simulink library "FoldingMechanisms"  (R2017a)
settings: Solver=VariableStepAuto  StartTime=0.0  StopTime=10.0  RelTol=1e-3
undefined symbols (not defined in the file or in its folder): X, Y, Z
libraries: sm_lib x70, FoldingMechanisms x62, nesl_utility x7
(part 1 of 4)
settings Model: Creator=merz  LastModifiedBy=Paris

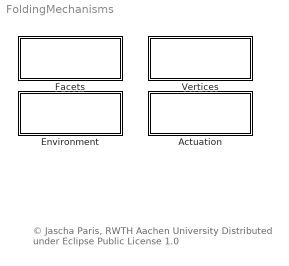
== system FoldingMechanisms ==
  note: © Jascha Paris, RWTH Aachen University
      |
      | Distributed under Eclipse Public License 1.0
  Actuation : Subsystem  Tag=FoldingMechanisms_sublibrary
      mask Display: disp(get_param(gcb,'Name'))
  Environment : Subsystem  Tag=FoldingMechanisms_sublibrary
      mask Display: disp(get_param(gcb,'Name'))
  Facets : Subsystem  Tag=FoldingMechanisms_sublibrary
      mask Display: disp(get_param(gcb,'Name'))
  Vertices : Subsystem  Tag=FoldingMechanisms_sublibrary
      mask Display: disp(get_param(gcb,'Name'))

== system FoldingMechanisms/Actuation ==
  Rotational Drive : Subsystem  mask{startang=1, endang=179, T_period=10, motion_select=sinus, forbac=on}
      mask prompts: startang "Start angle [°]"; endang "End angle [°]"; T_period "Periodic Time [s]"; motion_select "Motion Type"; forbac "Move forward and backward"
      mask init:
      | %Motion
      | startang_rad= startang*(pi/180);
      | endang_rad= endang*(pi/180);
      | steps=5000;
      | switch motion_select
      |     case 1
      |         t= [0,T_period/2]';
      |         y= [startang_rad,endang_rad]';
      |     case 2
      |         t= linspace(0,T_period/2,steps)';
      |         y= startang_rad+(endang_rad-startang_rad)*(1-(cos(linspace(0,pi,steps))'+1)/2);
      |     case 3
      |         t= linspace(0,T_period/2,steps)';
      |         z=t/(T_period/2);
      |         y=startang_rad+(endang_rad-startang_rad)*(6*z.^5-15*z.^4+10*z.^3);
      |     otherwise
      |         t= [0,T_period/2]';
      |         y= [startang_rad,endang_rad]';        
      | end
      | 
      | if (forbac==true)
      |     t= [t;t(2:end)+t(end)];
      |     y= [y;flipud(y(1:end-1))];    
      | end   
      |  
      | drivefunc = [t,y];
      mask TypeOptions motion_select: ramp | sinus | poly5
      mask DialogControl DescTextVar Prompt: This block provides, based on the parameters given below, a drive function for one foldangle of an actuated fold vertex
      mask Display:
      | plot([0.2 0.2], [0.2 0.8]);
      | plot([0.2 0.8], [0.2 0.2]);
      | 
      | scale_t=0.6/(max(t)-min(t));
      | scale_y=0.6/(max(y)-min(y));
      | 
      | plot(0.2+scale_t*(t-min(t)), 0.2+scale_y*(y-min(y)));

== system FoldingMechanisms/Environment ==
  Environment : Subsystem  Tag=simscape_sublibrary  mask{g_const=[0;0;-9.81]}
      mask prompts: g_const "Gravitational Constant"
      mask DialogControl DescTextVar Prompt: This Environment contains the local Simscape solver, gravity and the world coordinate system.
      mask Display: disp(get_param(gcb,'Name'))
  Options : Subsystem  Tag=simscape_sublibrary  mask{show3D=on}
      mask prompts: show3D "Show 3D Visualisation"
      mask Callback show3D:
      | show3D=get_param(gcb,'show3D');
      | mymodel=get_param(gcb,'parent');
      | if ~strcmp(mymodel,'FoldingMechanisms/Environment')
      |     if strcmp(show3D,'on');
      |         set_param(mymodel,'SimMechanicsOpenEditorOnUpdate','on');
      |     else
      |         set_param(mymodel,'SimMechanicsOpenEditorOnUpdate','off');
      |     end
      | end
      mask DialogControl DescTextVar Prompt: This block promotes options of the Simulation for convenience.
      mask Display: disp(get_param(gcb,'Name'))

== system FoldingMechanisms/Facets ==
  Piece of ellipsoid : Subsystem  Tag=simscape_sublibrary  mask{l1=0.4, l2=0.4, theta_x=35, tur1=off, tur2=off, t=0.01, clr=[200 200 200], tr=0.8, rjs1=on, rjs2=on, t_rj=0.01, cl_joint=[200 200 200]}
      mask prompts: l1 "Length S1 [m]"; l2 "Length S2 [m]"; theta_x "Angle alpha [°]"; tur1 "Turn COS at S1"; tur2 "Turn COS at S2"; t "Thickness [m]"; clr "Color RGB [3x1] with [0..255]"; tr "Transparency [0..1]"; rjs1 "at S1"; rjs2 "at S2"; t_rj "thickness"; cl_joint "Thickness [m]"
      mask init:
      | %Initialize Variables
      | a=0;
      | 
      | phi=linspace(0,theta_x,100);
      | r=linspace(l2,l1,100);
      | ellipsoid1=[r.*cosd(phi);r.*sind(phi)].';
      | 
      | %calculate geometry
      | cx=l1*cosd(theta_x);
      | cy=l1*sind(theta_x);
      | 
      | ellipsoid = [0 0; ellipsoid1];
      | 
      | bx=cx/2;
      | by=cy/2;
      | 
      | %Turn COS about 180° if enabled
      | turn1=0 + (tur1==true)*180;
      | turn2=0 + (tur2==true)*180;
      | 
      | %Convert color to vector with [0..1]
      | clr=clr/255;
      | cl_joint= cl_joint/255;
      | 
      | %Enable revolute joint visibility
      | %Convert logical to number
      | rj_true1=0 + (rjs1==true)*1;
      | rj_true2=0 + (rjs2==true)*1;
      mask DialogControl DescTextVar Prompt: Facet with two foldlines and an eliptic shape.
      mask DialogControl Container8 Prompt: Kinematic Dimensions
      mask DialogControl Container9 Prompt: Coordinate Systems
      mask DialogControl Control4 Prompt: Visualisation [on/off]
      mask Display:
      | %Geometry
      | X=[[0;0],ellipsoid1'];
      | 
      | %Normalized
      | dx=max(X(1,:))-min(X(1,:));
      | dy=max(X(2,:))-min(X(2,:));
      | dmax=max(dx,dy);
      | X=(X-[min(X(1,:));min(X(2,:))])/dmax*0.9+[0.05;0.05];
      | 
      | %Plot triangle
      | patch(X(1,:), X(2,:), clr);
      | plot([X(1,:),X(1,1)], [X(2,:),X(2,1)]);
      | 
      | 
      | %Labels in graphic
      | start_i=[1,1];
      | end_i=[size(X,2),2];
      | tur_f=[1,1];
      | 
      | color('blue');
      | for i=1:2
      |     if eval(['tur',num2str(i)])==tur_f(i)
      |         txt(i,1)='+';
      |         txt(i,2)='-';
      |     else
      |         txt(i,1)='-';
      |         txt(i,2)='+';
      |     end
      |     xs=X(1,start_i(i));
      |     vx=X(1,end_i(i))-X(1,start_i(i));
      |     ys=X(2,start_i(i));
      |     vy=X(2,end_i(i))-X(2,start_i(i));
      |     text(xs+vx*0.5,ys+vy*0.5,['S',num2str(i)]);
      |     text(xs+vx*0.3,ys+vy*0.3,txt(i,1));
      |     text(xs+vx*0.7,ys+vy*0.7,txt(i,2));
      | end
      | text((X(1,1)+X(1,end))/4,(X(2,1)+X(2,end))/7,'alpha');
  Quadrilateral : Subsystem  Tag=simscape_sublibrary  mask{l1=0.4, l2=0.4, l3=0.3, l4=0.5, alpha=80, tur1=off, tur2=off, tur3=off, tur4=off, t=0.01, clr=[200 200 200], tr=0.8, rjs1=on, rjs2=on, rjs3=on, rjs4=on, t_rj=0.01, cl_joint=[200 200 200]}
      mask prompts: l1 "Length S1 [m]"; l2 "Length S2 [m]"; l3 "Length S3 [m]"; l4 "Length S4 [m]"; alpha "Angle alpha [°]"; tur1 "Turn COS at S1"; tur2 "Turn COS at S2"; tur3 "Turn COS at S3"; tur4 "Turn COS at S4"; t "Thickness [m]"; clr "Color RGB [3x1] with [0..255]"; tr "Transparency [0..1]"; rjs1 "at S1"; rjs2 "at S2"; rjs3 "at S3"; rjs4 "at S4"; t_rj "Thickness [m]"; cl_joint "Color RGB [3x1] with [0..255]"
      mask init:
      | %Initialize Variables
      | a=0;
      | 
      | %calculate geometry
      | diagonal = sqrt(l1^2+l2^2-2*l1*l2*cosd(alpha));
      | 
      | a_x = 0;
      | a_y = 0;
      | b_x = l1*cosd(alpha);
      | b_y = l1*sind(alpha);
      | c_x = l2;
      | c_y = 0;
      | 
      | gamma1 = acosd((l2^2+diagonal^2-l1^2)/(2*l2*diagonal));
      | gamma2 = acosd((l3^2+diagonal^2-l4^2)/(2*l3*diagonal));
      | sigma = 180 - gamma1 - gamma2;
      | 
      | d_x = c_x + l3*cosd(sigma);
      | d_y = c_y + l3*sind(sigma);
      | 
      | ABmx = l1*cosd(alpha)/2;
      | ABmy = l1*sind(alpha)/2;
      | ACmx = l2/2;
      | ACmy = 0;
      | CDmx = c_x + l3*cosd(sigma)/2;
      | CDmy = c_y + l3*sind(sigma)/2;
      | 
      | beta1 = acosd((l1^2+diagonal^2-l2^2)/(2*l1*diagonal));
      | beta2 = acosd((l4^2+diagonal^2-l3^2)/(2*l4*diagonal));
      | epsilon = beta1 + beta2 + alpha - 180;
      | 
      | BDmx = b_x + l4*cosd(epsilon)/2;
      | BDmy = b_y + l4*sind(epsilon)/2;
      | 
      | quadrilateral=[b_x b_y; a_x a_y; c_x c_y; d_x d_y];
      | 
      | %Turn COS about 180° if enabled
      | turn1=0 + (tur1==true)*180;
      | turn2=0 + (tur2==true)*180;
      | turn3=0 + (tur3==true)*180;
      | turn4=0 + (tur4==true)*180;
      | 
      | %Convert color to vector with [0..1]
      | clr=clr/255;
      | cl_joint= cl_joint/255;
      | 
      | %Enable revolute joint visibility
      | %Convert logical to number
      | rj_true1=0 + (rjs1==true)*1;
      | rj_true2=0 + (rjs2==true)*1;
      | rj_true3=0 + (rjs3==true)*1;
      | rj_true4=0 + (rjs4==true)*1;
      mask DialogControl DescGroupVar Prompt: Quadrilateral Facet
      mask DialogControl DescTextVar Prompt: Facet with four foldlines.
      mask DialogControl Control3 Prompt: Visualisation [on/off]
      mask Display:
      | %Geometry
      | x_A=[a_x;a_y];
      | x_C=[c_x;c_y];
      | x_D=[d_x;d_y];
      | x_B=[b_x;b_y];
      | 
      | X=[x_A,x_C,x_D,x_B];
      | 
      | %Normalized
      | dx=max(X(1,:))-min(X(1,:));
      | dy=max(X(2,:))-min(X(2,:));
      | dmax=max(dx,dy);
      | X=(X-[min(X(1,:));min(X(2,:))])/dmax*0.9+[0.05;0.05];
      | 
      | %Plot Quadrilateral
      | patch(X(1,:), X(2,:), clr);
      | plot([X(1,:),X(1,1)], [X(2,:),X(2,1)]);
      | 
      | %Labels in graphic
      | color('blue');
      | 
      | start_i=[1,1,2,3];
      | end_i=[4,2,3,4];
      | tur_f=[1,1,1,0];
      | 
      | color('blue');
      | for i=1:4
      |     if eval(['tur',num2str(i)])==tur_f(i)
      |         txt(i,1)='+';
      |         txt(i,2)='-';
      |     else
      |         txt(i,1)='-';
      |         txt(i,2)='+';
      |     end
      |     xs=X(1,start_i(i));
      |     vx=X(1,end_i(i))-X(1,start_i(i));
      |     ys=X(2,start_i(i));
      |     vy=X(2,end_i(i))-X(2,start_i(i));
      |     text(xs+vx*0.5,ys+vy*0.5,['S',num2str(i)]);
      |     text(xs+vx*0.3,ys+vy*0.3,txt(i,1));
      |     text(xs+vx*0.7,ys+vy*0.7,txt(i,2));
      | end
      | text((X(1,1)+X(1,4))/4,(X(2,1)+X(2,4))/7,'alpha');
  Quintilateral : Subsystem  Tag=simscape_sublibrary  mask{l1=0.22, l2=0.13, l3=0.13, l4=0.27, l5=0.13, alpha=93, beta=120, tur1=off, tur2=off, tur3=off, tur4=off, tur5=off, thickness=0.01, clr=[200 200 200], tr=0.8, rjs1=on, rjs2=on, rjs3=on, rjs4=on, rjs5=on, t_rj=0.01, cl_joint=[200 200 200]}
      mask prompts: l1 "Length S1 [m]"; l2 "Length S2 [m]"; l3 "Length S3 [m]"; l4 "Length S4 [m]"; l5 "Length S5 [m]"; alpha "Angle alpha [°]"; beta "Angle beta [°]"; tur1 "Turn COS at S1"; tur2 "Turn COS at S2"; tur3 "Turn COS at S3"; tur4 "Turn COS at S4"; tur5 "Turn COS at S5"; thickness "Thickness [m]"; clr "Color RGB [3x1] with [0..255]"; tr "Transparency [0..1]"; rjs1 "at S1"; rjs2 "at S2"; rjs3 "at S3"; rjs4 "at S4"; rjs5 "at S5"; t_rj "Thickness [m]"; cl_joint "Color RGB [3x1] with [0..255]"
      mask init:
      | %Given Points
      | a_x = 0;
      | a_y = 0;
      | b_x = l2;
      | b_y = 0;
      | c_x = b_x+l3*cosd(180-beta);
      | c_y = b_y+l3*sind(180-beta);
      | e_x = l1*cosd(alpha);
      | e_y = l1*sind(alpha);
      | 
      | %calculate geometry
      | Dx=e_x-c_x;
      | Dy=e_y-c_y;
      | la=-l5;
      | lb=l4;
      | Calpha=(Dx^2+Dy^2+la^2-lb^2)/(2*la);
      | t=(Dy-sqrt(Dx^2+Dy^2-Calpha^2))/(Dx+Calpha);
      | talpha=2*atand(t);
      | Cbeta=(Dx^2+Dy^2+lb^2-la^2)/(2*lb);
      | tb=(Dy-sqrt(Dx^2+Dy^2-Cbeta^2))/(Dx+Cbeta);
      | tbeta=2*atand(tb);
      | d_x=e_x+(1-t^2)/(1+t^2)*l5;
      | d_y=e_y+(2*t)/(1+t^2)*l5;
      | 
      | quadrilateral=[a_x a_y; b_x b_y; c_x c_y; d_x d_y; e_x e_y];
      | 
      | %Turn COS about 180° if enabled
      | turn1=0 + (tur1==true)*180;
      | turn2=0 + (tur2==true)*180;
      | turn3=0 + (tur3==true)*180;
      | turn4=0 + (tur4==true)*180;
      | turn5=0 + (tur5==true)*180;
      | 
      | %Convert color to vector with [0..1]
      | clr=clr/255;
      | cl_joint= cl_joint/255;
      | 
      | %Enable revolute joint visibility
      | %Convert logical to number
      | rj_true1=0 + (rjs1==true)*1;
      | rj_true2=0 + (rjs2==true)*1;
      | rj_true3=0 + (rjs3==true)*1;
      | rj_true4=0 + (rjs4==true)*1;
      | rj_true5=0 + (rjs5==true)*1;
      mask DialogControl DescGroupVar Prompt: Quadrilateral Facet
      mask DialogControl DescTextVar Prompt: Facet with four foldlines.
      mask DialogControl Control3 Prompt: Visualisation [on/off]
      mask Display:
      | %Geometry
      | 
      | X=quadrilateral.';
      | 
      | %Normalized
      | dx=max(X(1,:))-min(X(1,:));
      | dy=max(X(2,:))-min(X(2,:));
      | dmax=max(dx,dy);
      | X=(X-[min(X(1,:));min(X(2,:))])/dmax*0.9+[0.05;0.05];
      | 
      | %Plot Quadrilateral
      | patch(X(1,:), X(2,:), clr);
      | plot([X(1,:),X(1,1)], [X(2,:),X(2,1)]);
      | 
      | 
      | %Labels in graphic
      | color('blue');
      | 
      | start_i=[1,1,2,3,4];
      | end_i=[5,2,3,4,5];
      | tur_f=[1,1,1,0,0];
      | 
      | color('blue');
      | for i=1:5
      |     if eval(['tur',num2str(i)])==tur_f(i)
      |         txt(i,1)='+';
      |         txt(i,2)='-';
      |     else
      |         txt(i,1)='-';
      |         txt(i,2)='+';
      |     end
      |     xs=X(1,start_i(i));
      |     vx=X(1,end_i(i))-X(1,start_i(i));
      |     ys=X(2,start_i(i));
      |     vy=X(2,end_i(i))-X(2,start_i(i));
      |     text(xs+vx*0.5,ys+vy*0.5,['S',num2str(i)]);
      |     text(xs+vx*0.3,ys+vy*0.3,txt(i,1));
      |     text(xs+vx*0.7,ys+vy*0.7,txt(i,2));
      | end
      | text((X(1,1)+X(1,2))/4,(X(2,1)+X(2,2))/2+0.06,'alpha');
      | text((X(1,1)+X(1,2))*3/4,(X(2,1)+X(2,2))/2+0.06,'beta');
  Triangle : Subsystem  Tag=simscape_sublibrary  mask{l1=0.4, l2=0.4, alpha=60, tur1=off, tur2=off, tur3=off, t=0.01, clr=[200 200 200], tr=0.8, rjs1=on, rjs2=on, rjs3=on, t_rj=0.01, cl_joint=[200 200 200]}
      mask prompts: l1 "Length S1 [m]"; l2 "Length S3 [m]"; alpha "Angle alpha [°]"; tur1 "Turn COS at S1"; tur2 "Turn COS at S2"; tur3 "Turn COS at S3"; t "Thickness [m]"; clr "Color RGB [3x1] with [0..255]"; tr "Transparency [0..1]"; rjs1 "at S1"; rjs2 "at S2"; rjs3 "at S3"; t_rj "Thickness [m]"; cl_joint "Color RGB [3x1] with [0..255]"
      mask init:
      | %Initialize Variables
      | a=0;
      | p=1;
      | 
      | %Calculate geometry
      | w1 = -l2/2 + l1*cosd(alpha);
      | h1 = p*(l1*sind(alpha));
      | l3 = sqrt(l1^2 + l2^2 - 2*l1*l2*cosd(alpha));
      | beta = acosd((l3^2+l2^2-l1^2)/(2*l3*l2));
      | w2 = -l2/2 + l1*cosd(alpha)/2;
      | w3 = l2/2 - l3*cosd(beta)/2;
      | h2 = (h1/2);
      | triangle= [w1 h1; p*(-l2/2) 0; p*(l2/2) 0];
      | 
      | %Turn COS about 180° if enabled
      | turn1=0 + (tur1==true)*180;
      | turn2=0 + (tur2==true)*180;
      | turn3=0 + (tur3==true)*180;
      | 
      | %Convert color to vector with [0..1]
      | clr=clr/255;
      | cl_joint= cl_joint/255;
      | 
      | %Enable revolute joint visibility
      | %Convert logical to number
      | rj_true1=0 + (rjs1==true)*1;
      | rj_true2=0 + (rjs2==true)*1;
      | rj_true3=0 + (rjs3==true)*1;
      mask DialogControl DescGroupVar Prompt: Triangular Facet
      mask DialogControl DescTextVar Prompt: Facet with three foldlines.
      mask DialogControl txt_rev Prompt: Visualisation [on/off]
      mask Display:
      | %Prepare visualisation of triangle
      | X=triangle';
      | 
      | %Normalize triangle
      | dx=max(X(1,:))-min(X(1,:));
      | dy=max(X(2,:))-min(X(2,:));
      | dmax=max(dx,dy);
      | X=(X-[min(X(1,:));min(X(2,:))])/dmax*0.9+[0.05;0.05];
      | 
      | %Plot triangle
      | patch(X(1,:), X(2,:), clr);
      | plot([X(1,:),X(1,1)], [X(2,:),X(2,1)]);
      | 
      | 
      | %Labels in graphic
      | 
      | start_i=[1,1,2];
      | end_i=[2,3,3];
      | tur_f=[0,0,1];
      | 
      | color('blue');
      | for i=1:3
      |     if eval(['tur',num2str(i)])==tur_f(i)
      |         txt(i,1)='+';
      |         txt(i,2)='-';
      |     else
      |         txt(i,1)='-';
      |         txt(i,2)='+';
      |     end
      |     xs=X(1,start_i(i));
      |     vx=X(1,end_i(i))-X(1,start_i(i));
      |     ys=X(2,start_i(i));
      |     vy=X(2,end_i(i))-X(2,start_i(i));
      |     text(xs+vx*0.5,ys+vy*0.5,['S',num2str(i)]);
      |     text(xs+vx*0.3,ys+vy*0.3,txt(i,1));
      |     text(xs+vx*0.7,ys+vy*0.7,txt(i,2));
      | end
      | text((X(1,1)+X(1,2))/4,(X(2,1)+X(2,2))/7,'alpha');

== system FoldingMechanisms/Vertices ==
  4-Foldlines Vertices : Subsystem  Tag=simscape_sublibrary
      mask Display: disp(get_param(gcb,'Name'))
  5-Foldlines Vertices : Subsystem  Tag=simscape_sublibrary
      mask Display: disp(get_param(gcb,'Name'))
  6-Foldlines Vertices : Subsystem  Tag=simscape_sublibrary
      mask Display: disp(get_param(gcb,'Name'))
  7-Foldlines Vertices : Subsystem  Tag=simscape_sublibrary
      mask Display: disp(get_param(gcb,'Name'))
  8-Foldlines Vertices : Subsystem  Tag=simscape_sublibrary
      mask Display: disp(get_param(gcb,'Name'))
  Subelements : Subsystem  Tag=simscape_sublibrary
      mask Display: disp(get_param(gcb,'Name'))

== system FoldingMechanisms/Actuation/Rotational Drive ==
  From Workspace : FromWorkspace  VariableName=drivefunc  SampleTime=0  OutputAfterFinalValue=Holding final value
  Drive Function : Outport
  wires:
  From Workspace/1 -> Drive Function/1

== system FoldingMechanisms/Environment/Environment ==
  Mechanism Configuration : sm_lib/Utilities/Mechanism Configuration  UniformGravity=Constant  GravityVector=g_const  GravityUnits=m/s^2  LinearizationDelta=0.001
  Solver Configuration : nesl_utility/Solver Configuration  PhysicalDomain=network_engine_domain  SubClassName=solver  LeftPortType=input  RightPortType=generic  Accelerate=off  Tones=[]  Harmonics=[]  SimulateNoise=off  Profile=off  UseLocalSampling=off  EnableSwitchedLinearOptims=on  FrequencyDomain=off  UseCCode=off  RelTol=0.001  AbsTol=1e-06  MinStep=1e-09  ToWorkspace=off  RevertToSquareIcSolve=off  NumHomotopyIterations=100  PhasorMode=off  PhasorModeNumHarmonics=1  OverrideAbsTol=off  DoDC=off  ResidualTolerance=1e-09  UseLocalSolver=off  LocalSolverChoice=NE_BACKWARD_EULER_ADVANCER  LocalSolverSampleTime=0.001  DoFixedCost=off  MaxNonlinIter=3  MaxModeIter=2  LinearAlgebra=Sparse  DelaysMemoryBudget=1024  AutomaticFiltering=on  FilteringTimeConstant=0.001
  World Frame : sm_lib/Frames and Transforms/World Frame
  Environment Port : PMIOPort  Port=1  Side=Right
  connections:
  Mechanism Configuration/RConn1 -- Environment Port/RConn1 -- World Frame/RConn1 -- Solver Configuration/RConn1

== system FoldingMechanisms/Environment/Options ==

== system FoldingMechanisms/Facets/Piece of ellipsoid ==
  Rigid Transform 1.1 : sm_lib/Frames and Transforms/Rigid Transform  TranslationMethod=Cartesian  TranslationStandardOffset=0  TranslationLengthUnit=m  TranslationStandardAxis=+Z  TranslationCartesianOffset=[bx by 0]  TranslationROffset=0  TranslationROffsetUnits=m  TranslationZOffset=0  TranslationZOffsetUnits=m  TranslationThetaOffset=0  TranslationThetaOffsetUnits=deg  RotationMethod=None  RotationAngleUnits=deg  RotationStandardAxis=+Z  RotationAngle=0.0  RotationArbitraryAxis=[0 0 1]  FollAlignAxisA=+X  BaseAlignAxisA=+Y  FollAlignAxisB=+Y  BaseAlignAxisB=+Z  RotationSequenceAxes=FollowerAxes  RotationSequence=XYX  RotationSequenceAngles=[0 0 0]  RotationSequenceAnglesUnits=deg  RotationMatrix=[1 0 0; 0 1 0; 0 0 1]
  Rigid Transform 1.2 : sm_lib/Frames and Transforms/Rigid Transform  TranslationMethod=None  TranslationStandardOffset=0  TranslationLengthUnit=m  TranslationStandardAxis=+Z  TranslationCartesianOffset=[0 0 0]  TranslationROffset=0  TranslationROffsetUnits=m  TranslationZOffset=0  TranslationZOffsetUnits=m  TranslationThetaOffset=0  TranslationThetaOffsetUnits=deg  RotationMethod=StandardAxis  RotationAngleUnits=deg  RotationStandardAxis=+Z  RotationAngle=theta_x  RotationArbitraryAxis=[0 0 1]  FollAlignAxisA=+X  BaseAlignAxisA=+Y  FollAlignAxisB=+Y  BaseAlignAxisB=+Z  RotationSequenceAxes=FollowerAxes  RotationSequence=XYX  RotationSequenceAngles=[0 0 0]  RotationSequenceAnglesUnits=deg  RotationMatrix=[1 0 0; 0 1 0; 0 0 1]
  Rigid Transform 1.3 : sm_lib/Frames and Transforms/Rigid Transform  TranslationMethod=None  TranslationStandardOffset=0  TranslationLengthUnit=m  TranslationStandardAxis=+Z  TranslationCartesianOffset=[0 0 0]  TranslationROffset=0  TranslationROffsetUnits=m  TranslationZOffset=0  TranslationZOffsetUnits=m  TranslationThetaOffset=0  TranslationThetaOffsetUnits=deg  RotationMethod=StandardAxis  RotationAngleUnits=deg  RotationStandardAxis=+Y  RotationAngle=90  RotationArbitraryAxis=[0 0 1]  FollAlignAxisA=+X  BaseAlignAxisA=+Y  FollAlignAxisB=+Y  BaseAlignAxisB=+Z  RotationSequenceAxes=FollowerAxes  RotationSequence=XYX  RotationSequenceAngles=[0 0 0]  RotationSequenceAnglesUnits=deg  RotationMatrix=[1 0 0; 0 1 0; 0 0 1]
  Rigid Transform 1.4 : sm_lib/Frames and Transforms/Rigid Transform  TranslationMethod=None  TranslationStandardOffset=0  TranslationLengthUnit=m  TranslationStandardAxis=+Z  TranslationCartesianOffset=[0 0 0]  TranslationROffset=0  TranslationROffsetUnits=m  TranslationZOffset=0  TranslationZOffsetUnits=m  TranslationThetaOffset=0  TranslationThetaOffsetUnits=deg  RotationMethod=StandardAxis  RotationAngleUnits=deg  RotationStandardAxis=+X  RotationAngle=turn1  RotationArbitraryAxis=[0 0 1]  FollAlignAxisA=+X  BaseAlignAxisA=+Y  FollAlignAxisB=+Y  BaseAlignAxisB=+Z  RotationSequenceAxes=FollowerAxes  RotationSequence=XYX  RotationSequenceAngles=[0 0 0]  RotationSequenceAnglesUnits=deg  RotationMatrix=[1 0 0; 0 1 0; 0 0 1]
  Rigid Transform 2.1 : sm_lib/Frames and Transforms/Rigid Transform  TranslationMethod=Cartesian  TranslationStandardOffset=0  TranslationLengthUnit=m  TranslationStandardAxis=+Z  TranslationCartesianOffset=[l2/2 0 0]  TranslationROffset=0  TranslationROffsetUnits=m  TranslationZOffset=0  TranslationZOffsetUnits=m  TranslationThetaOffset=0  TranslationThetaOffsetUnits=deg  RotationMethod=StandardAxis  RotationAngleUnits=deg  RotationStandardAxis=+Y  RotationAngle=90  RotationArbitraryAxis=[0 0 1]  FollAlignAxisA=+X  BaseAlignAxisA=+Y  FollAlignAxisB=+Y  BaseAlignAxisB=+Z  RotationSequenceAxes=FollowerAxes  RotationSequence=XYX  RotationSequenceAngles=[0 0 0]  RotationSequenceAnglesUnits=deg  RotationMatrix=[1 0 0; 0 1 0; 0 0 1]
  Rigid Transform 2.2 : sm_lib/Frames and Transforms/Rigid Transform  TranslationMethod=None  TranslationStandardOffset=0  TranslationLengthUnit=m  TranslationStandardAxis=+Z  TranslationCartesianOffset=[0 0 0]  TranslationROffset=0  TranslationROffsetUnits=m  TranslationZOffset=0  TranslationZOffsetUnits=m  TranslationThetaOffset=0  TranslationThetaOffsetUnits=deg  RotationMethod=StandardAxis  RotationAngleUnits=deg  RotationStandardAxis=+X  RotationAngle=turn2  RotationArbitraryAxis=[0 0 1]  FollAlignAxisA=+X  BaseAlignAxisA=+Y  FollAlignAxisB=+Y  BaseAlignAxisB=+Z  RotationSequenceAxes=FollowerAxes  RotationSequence=XYX  RotationSequenceAngles=[0 0 0]  RotationSequenceAnglesUnits=deg  RotationMatrix=[1 0 0; 0 1 0; 0 0 1]
  Solid_RJ1 : sm_lib/Body Elements/Solid  InertiaType=PointMass  Mass=0  MassUnits=kg  CenterOfMass=[0 0 0]  CenterOfMassUnits=m  MomentsOfInertia=[1 1 1]  MomentsOfInertiaUnits=kg*m^2  ProductsOfInertia=[1 1 1]  ProductsOfInertiaUnits=kg*m^2  DensityBased=on  Density=1000  DensityUnits=kg/m^3  DoExposeReferenceFrame=off  SerializedFrames=<Frames><Frame><Id>Frame1</Id><Value><Name>S1</Name><Origin><Source>ReferenceFrame</Source><FeatureName></FeatureName></Origin><PrimaryAxis><DefinedDirection>+Z</DefinedDirection><Source>ReferenceFrame</Source><SourceDirection>+Z</SourceDirection><FeatureName></FeatureName></PrimaryAxis><SecondaryAxis><DefinedDirection>+X</DefinedDirection><Source>ReferenceFrame</Source><SourceDirection>+X</SourceDirection><FeatureName></FeatureName></SecondaryAxis></Value></Frame></Frames>  GraphicType=FromGeometry  MarkerShape=Sphere  MarkerSize=10  GraphicVisPropType=SimpleVisualProperties  GraphicDiffuseColor=cl_joint  GraphicSpecularColor=[0.5 0.5 0.5 1.0]  GraphicAmbientColor=[0.15 0.15 0.15 1.0]  GraphicEmissiveColor=[0.0 0.0 0.0 1.0]  GraphicShininess=75  GraphicOpacity=rj_true1  GeometryShape=Cylinder  RectangleSize=[1 1]  RectangleSizeUnits=m  BrickDimensions=[1 1 1]  BrickDimensionUnits=m  CylinderRadius=t_rj  CylinderRadiusUnits=m  CylinderLength=l1  CylinderLengthUnits=m  SphereRadius=1  SphereRadiusUnits=m  EllipsoidRadii=[1 1 1]  EllipsoidRadiiUnits=m  ExtrusionCrossSection=[1 1; -1 1; -1 -1; 1 -1]  ExtrusionCrossSectionUnits=m  ExtrusionLength=1  ExtrusionLengthUnits=m  PolygonNumSides=3  PolygonOuterRadius=1  PolygonOuterRadiusUnits=m  ExtGeomFileType=STEP  ExtGeomFileUnits=m  RevolutionCrossSection=[1 1; 1 -1; 2 -1; 2 1]  RevolutionCrossSectionUnits=m  RevolutionExtent=Full  RevolutionAngle=180  RevolutionAngleUnits=deg
  Solid_RJ2 : sm_lib/Body Elements/Solid  InertiaType=PointMass  Mass=0  MassUnits=kg  CenterOfMass=[0 0 0]  CenterOfMassUnits=m  MomentsOfInertia=[1 1 1]  MomentsOfInertiaUnits=kg*m^2  ProductsOfInertia=[1 1 1]  ProductsOfInertiaUnits=kg*m^2  DensityBased=on  Density=1000  DensityUnits=kg/m^3  DoExposeReferenceFrame=off  SerializedFrames=<Frames><Frame><Id>Frame1</Id><Value><Name>S2</Name><Origin><Source>ReferenceFrame</Source><FeatureName></FeatureName></Origin><PrimaryAxis><DefinedDirection>+Z</DefinedDirection><Source>ReferenceFrame</Source><SourceDirection>+Z</SourceDirection><FeatureName></FeatureName></PrimaryAxis><SecondaryAxis><DefinedDirection>+X</DefinedDirection><Source>ReferenceFrame</Source><SourceDirection>+X</SourceDirection><FeatureName></FeatureName></SecondaryAxis></Value></Frame></Frames>  GraphicType=FromGeometry  MarkerShape=Sphere  MarkerSize=10  GraphicVisPropType=SimpleVisualProperties  GraphicDiffuseColor=cl_joint  GraphicSpecularColor=[0.5 0.5 0.5 1.0]  GraphicAmbientColor=[0.15 0.15 0.15 1.0]  GraphicEmissiveColor=[0.0 0.0 0.0 1.0]  GraphicShininess=75  GraphicOpacity=rj_true2  GeometryShape=Cylinder  RectangleSize=[1 1]  RectangleSizeUnits=m  BrickDimensions=[1 1 1]  BrickDimensionUnits=m  CylinderRadius=t_rj  CylinderRadiusUnits=m  CylinderLength=l2  CylinderLengthUnits=m  SphereRadius=1  SphereRadiusUnits=m  EllipsoidRadii=[1 1 1]  EllipsoidRadiiUnits=m  ExtrusionCrossSection=[1 1; -1 1; -1 -1; 1 -1]  ExtrusionCrossSectionUnits=m  ExtrusionLength=1  ExtrusionLengthUnits=m  PolygonNumSides=3  PolygonOuterRadius=1  PolygonOuterRadiusUnits=m  ExtGeomFileType=STEP  ExtGeomFileUnits=m  RevolutionCrossSection=[1 1; 1 -1; 2 -1; 2 1]  RevolutionCrossSectionUnits=m  RevolutionExtent=Full  RevolutionAngle=180  RevolutionAngleUnits=deg
  Solid_ellipsoid : sm_lib/Body Elements/Solid  InertiaType=CalculateFromGeometry  Mass=1  MassUnits=kg  CenterOfMass=[0 0 0]  CenterOfMassUnits=m  MomentsOfInertia=[1 1 1]  MomentsOfInertiaUnits=kg*m^2  ProductsOfInertia=[1 1 1]  ProductsOfInertiaUnits=kg*m^2  DensityBased=on  Density=1000  DensityUnits=kg/m^3  DoExposeReferenceFrame=on  SerializedFrames=<Frames/>  GraphicType=FromGeometry  MarkerShape=Sphere  MarkerSize=10  GraphicVisPropType=SimpleVisualProperties  GraphicDiffuseColor=clr  GraphicSpecularColor=[0.5 0.5 0.5 1.0]  GraphicAmbientColor=[0.15 0.15 0.15 1.0]  GraphicEmissiveColor=[0.0 0.0 0.0 1.0]  GraphicShininess=75  GraphicOpacity=tr  GeometryShape=GeneralExtrusion  RectangleSize=[1 1]  RectangleSizeUnits=m  BrickDimensions=[1 1 1]  BrickDimensionUnits=m  CylinderRadius=1  CylinderRadiusUnits=m  CylinderLength=1  CylinderLengthUnits=m  SphereRadius=1  SphereRadiusUnits=m  EllipsoidRadii=[1 1 1]  EllipsoidRadiiUnits=m  ExtrusionCrossSection=ellipsoid  ExtrusionCrossSectionUnits=m  ExtrusionLength=t  ExtrusionLengthUnits=m  PolygonNumSides=3  PolygonOuterRadius=1  PolygonOuterRadiusUnits=m  ExtGeomFileType=STEP  ExtGeomFileUnits=m  RevolutionCrossSection=[1 1; 1 -1; 2 -1; 2 1]  RevolutionCrossSectionUnits=m  RevolutionExtent=Full  RevolutionAngle=180  RevolutionAngleUnits=deg
  S1 : PMIOPort  Port=1  Side=Left
  S2 : PMIOPort  Port=2  Side=Right
  connections:
  Rigid Transform 2.2/LConn1 -- Rigid Transform 2.1/RConn1
  Rigid Transform 1.3/RConn1 -- Rigid Transform 1.4/LConn1
  Rigid Transform 1.3/LConn1 -- Rigid Transform 1.2/RConn1
  Rigid Transform 1.2/LConn1 -- Rigid Transform 1.1/RConn1
  Solid_ellipsoid/RConn1 -- Rigid Transform 2.1/LConn1 -- Rigid Transform 1.1/LConn1
  S2/RConn1 -- Solid_RJ2/LConn1 -- Rigid Transform 2.2/RConn1
  S1/RConn1 -- Solid_RJ1/LConn1 -- Rigid Transform 1.4/RConn1

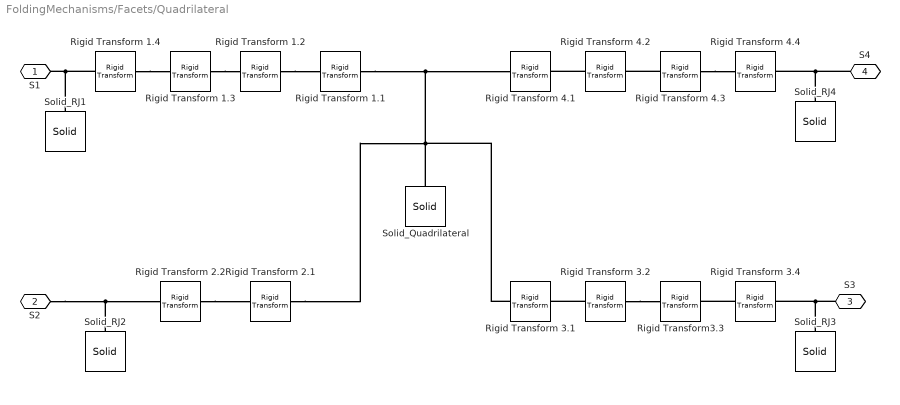
== system FoldingMechanisms/Facets/Quadrilateral ==
  Rigid Transform 1.1 : sm_lib/Frames and Transforms/Rigid Transform  TranslationMethod=Cartesian  TranslationStandardOffset=0  TranslationLengthUnit=m  TranslationStandardAxis=+Z  TranslationCartesianOffset=[ABmx ABmy 0]  TranslationROffset=0  TranslationROffsetUnits=m  TranslationZOffset=0  TranslationZOffsetUnits=m  TranslationThetaOffset=0  TranslationThetaOffsetUnits=deg  RotationMethod=None  RotationAngleUnits=deg  RotationStandardAxis=+Z  RotationAngle=0.0  RotationArbitraryAxis=[0 0 1]  FollAlignAxisA=+X  BaseAlignAxisA=+Y  FollAlignAxisB=+Y  BaseAlignAxisB=+Z  RotationSequenceAxes=FollowerAxes  RotationSequence=XYX  RotationSequenceAngles=[0 0 0]  RotationSequenceAnglesUnits=deg  RotationMatrix=[1 0 0; 0 1 0; 0 0 1]
  Rigid Transform 1.2 : sm_lib/Frames and Transforms/Rigid Transform  TranslationMethod=None  TranslationStandardOffset=0  TranslationLengthUnit=m  TranslationStandardAxis=+Z  TranslationCartesianOffset=[0 0 0]  TranslationROffset=0  TranslationROffsetUnits=m  TranslationZOffset=0  TranslationZOffsetUnits=m  TranslationThetaOffset=0  TranslationThetaOffsetUnits=deg  RotationMethod=StandardAxis  RotationAngleUnits=deg  RotationStandardAxis=+Z  RotationAngle=alpha  RotationArbitraryAxis=[0 0 1]  FollAlignAxisA=+X  BaseAlignAxisA=+Y  FollAlignAxisB=+Y  BaseAlignAxisB=+Z  RotationSequenceAxes=FollowerAxes  RotationSequence=XYX  RotationSequenceAngles=[0 0 0]  RotationSequenceAnglesUnits=deg  RotationMatrix=[1 0 0; 0 1 0; 0 0 1]
  Rigid Transform 1.3 : sm_lib/Frames and Transforms/Rigid Transform  TranslationMethod=Cartesian  TranslationStandardOffset=0  TranslationLengthUnit=m  TranslationStandardAxis=+Z  TranslationCartesianOffset=[0 a 0]  TranslationROffset=0  TranslationROffsetUnits=m  TranslationZOffset=0  TranslationZOffsetUnits=m  TranslationThetaOffset=0  TranslationThetaOffsetUnits=deg  RotationMethod=StandardAxis  RotationAngleUnits=deg  RotationStandardAxis=+Y  RotationAngle=90  RotationArbitraryAxis=[0 0 1]  FollAlignAxisA=+X  BaseAlignAxisA=+Y  FollAlignAxisB=+Y  BaseAlignAxisB=+Z  RotationSequenceAxes=FollowerAxes  RotationSequence=XYX  RotationSequenceAngles=[0 0 0]  RotationSequenceAnglesUnits=deg  RotationMatrix=[1 0 0; 0 1 0; 0 0 1]
  Rigid Transform 1.4 : sm_lib/Frames and Transforms/Rigid Transform  TranslationMethod=None  TranslationStandardOffset=0  TranslationLengthUnit=m  TranslationStandardAxis=+Z  TranslationCartesianOffset=[0 0 0]  TranslationROffset=0  TranslationROffsetUnits=m  TranslationZOffset=0  TranslationZOffsetUnits=m  TranslationThetaOffset=0  TranslationThetaOffsetUnits=deg  RotationMethod=StandardAxis  RotationAngleUnits=deg  RotationStandardAxis=+X  RotationAngle=turn1  RotationArbitraryAxis=[0 0 1]  FollAlignAxisA=+X  BaseAlignAxisA=+Y  FollAlignAxisB=+Y  BaseAlignAxisB=+Z  RotationSequenceAxes=FollowerAxes  RotationSequence=XYX  RotationSequenceAngles=[0 0 0]  RotationSequenceAnglesUnits=deg  RotationMatrix=[1 0 0; 0 1 0; 0 0 1]
  Rigid Transform 2.1 : sm_lib/Frames and Transforms/Rigid Transform  TranslationMethod=Cartesian  TranslationStandardOffset=0  TranslationLengthUnit=m  TranslationStandardAxis=+Z  TranslationCartesianOffset=[ACmx ACmy 0]  TranslationROffset=0  TranslationROffsetUnits=m  TranslationZOffset=0  TranslationZOffsetUnits=m  TranslationThetaOffset=0  TranslationThetaOffsetUnits=deg  RotationMethod=StandardAxis  RotationAngleUnits=deg  RotationStandardAxis=+Y  RotationAngle=90  RotationArbitraryAxis=[0 0 1]  FollAlignAxisA=+X  BaseAlignAxisA=+Y  FollAlignAxisB=+Y  BaseAlignAxisB=+Z  RotationSequenceAxes=FollowerAxes  RotationSequence=XYX  RotationSequenceAngles=[0 0 0]  RotationSequenceAnglesUnits=deg  RotationMatrix=[1 0 0; 0 1 0; 0 0 1]
  Rigid Transform 2.2 : sm_lib/Frames and Transforms/Rigid Transform  TranslationMethod=None  TranslationStandardOffset=0  TranslationLengthUnit=m  TranslationStandardAxis=+Z  TranslationCartesianOffset=[0 0 0]  TranslationROffset=0  TranslationROffsetUnits=m  TranslationZOffset=0  TranslationZOffsetUnits=m  TranslationThetaOffset=0  TranslationThetaOffsetUnits=deg  RotationMethod=StandardAxis  RotationAngleUnits=deg  RotationStandardAxis=+X  RotationAngle=turn2  RotationArbitraryAxis=[0 0 1]  FollAlignAxisA=+X  BaseAlignAxisA=+Y  FollAlignAxisB=+Y  BaseAlignAxisB=+Z  RotationSequenceAxes=FollowerAxes  RotationSequence=XYX  RotationSequenceAngles=[0 0 0]  RotationSequenceAnglesUnits=deg  RotationMatrix=[1 0 0; 0 1 0; 0 0 1]
  Rigid Transform 3.1 : sm_lib/Frames and Transforms/Rigid Transform  TranslationMethod=Cartesian  TranslationStandardOffset=0  TranslationLengthUnit=m  TranslationStandardAxis=+Z  TranslationCartesianOffset=[CDmx CDmy 0]  TranslationROffset=0  TranslationROffsetUnits=m  TranslationZOffset=0  TranslationZOffsetUnits=m  TranslationThetaOffset=0  TranslationThetaOffsetUnits=deg  RotationMethod=None  RotationAngleUnits=deg  RotationStandardAxis=+Z  RotationAngle=0.0  RotationArbitraryAxis=[0 0 1]  FollAlignAxisA=+X  BaseAlignAxisA=+Y  FollAlignAxisB=+Y  BaseAlignAxisB=+Z  RotationSequenceAxes=FollowerAxes  RotationSequence=XYX  RotationSequenceAngles=[0 0 0]  RotationSequenceAnglesUnits=deg  RotationMatrix=[1 0 0; 0 1 0; 0 0 1]
  Rigid Transform 3.2 : sm_lib/Frames and Transforms/Rigid Transform  TranslationMethod=None  TranslationStandardOffset=0  TranslationLengthUnit=m  TranslationStandardAxis=+Z  TranslationCartesianOffset=[0 0 0]  TranslationROffset=0  TranslationROffsetUnits=m  TranslationZOffset=0  TranslationZOffsetUnits=m  TranslationThetaOffset=0  TranslationThetaOffsetUnits=deg  RotationMethod=StandardAxis  RotationAngleUnits=deg  RotationStandardAxis=+Z  RotationAngle=sigma  RotationArbitraryAxis=[0 0 1]  FollAlignAxisA=+X  BaseAlignAxisA=+Y  FollAlignAxisB=+Y  BaseAlignAxisB=+Z  RotationSequenceAxes=FollowerAxes  RotationSequence=XYX  RotationSequenceAngles=[0 0 0]  RotationSequenceAnglesUnits=deg  RotationMatrix=[1 0 0; 0 1 0; 0 0 1]
  Rigid Transform 3.4 : sm_lib/Frames and Transforms/Rigid Transform  TranslationMethod=None  TranslationStandardOffset=0  TranslationLengthUnit=m  TranslationStandardAxis=+Z  TranslationCartesianOffset=[0 0 0]  TranslationROffset=0  TranslationROffsetUnits=m  TranslationZOffset=0  TranslationZOffsetUnits=m  TranslationThetaOffset=0  TranslationThetaOffsetUnits=deg  RotationMethod=StandardAxis  RotationAngleUnits=deg  RotationStandardAxis=+X  RotationAngle=turn3  RotationArbitraryAxis=[0 0 1]  FollAlignAxisA=+X  BaseAlignAxisA=+Y  FollAlignAxisB=+Y  BaseAlignAxisB=+Z  RotationSequenceAxes=FollowerAxes  RotationSequence=XYX  RotationSequenceAngles=[0 0 0]  RotationSequenceAnglesUnits=deg  RotationMatrix=[1 0 0; 0 1 0; 0 0 1]
  Rigid Transform 4.1 : sm_lib/Frames and Transforms/Rigid Transform  TranslationMethod=Cartesian  TranslationStandardOffset=0  TranslationLengthUnit=m  TranslationStandardAxis=+Z  TranslationCartesianOffset=[BDmx BDmy 0]  TranslationROffset=0  TranslationROffsetUnits=m  TranslationZOffset=0  TranslationZOffsetUnits=m  TranslationThetaOffset=0  TranslationThetaOffsetUnits=deg  RotationMethod=None  RotationAngleUnits=deg  RotationStandardAxis=+Z  RotationAngle=0.0  RotationArbitraryAxis=[0 0 1]  FollAlignAxisA=+X  BaseAlignAxisA=+Y  FollAlignAxisB=+Y  BaseAlignAxisB=+Z  RotationSequenceAxes=FollowerAxes  RotationSequence=XYX  RotationSequenceAngles=[0 0 0]  RotationSequenceAnglesUnits=deg  RotationMatrix=[1 0 0; 0 1 0; 0 0 1]
  Rigid Transform 4.2 : sm_lib/Frames and Transforms/Rigid Transform  TranslationMethod=None  TranslationStandardOffset=0  TranslationLengthUnit=m  TranslationStandardAxis=+Z  TranslationCartesianOffset=[0 0 0]  TranslationROffset=0  TranslationROffsetUnits=m  TranslationZOffset=0  TranslationZOffsetUnits=m  TranslationThetaOffset=0  TranslationThetaOffsetUnits=deg  RotationMethod=StandardAxis  RotationAngleUnits=deg  RotationStandardAxis=+Z  RotationAngle=epsilon  RotationArbitraryAxis=[0 0 1]  FollAlignAxisA=+X  BaseAlignAxisA=+Y  FollAlignAxisB=+Y  BaseAlignAxisB=+Z  RotationSequenceAxes=FollowerAxes  RotationSequence=XYX  RotationSequenceAngles=[0 0 0]  RotationSequenceAnglesUnits=deg  RotationMatrix=[1 0 0; 0 1 0; 0 0 1]
  Rigid Transform 4.3 : sm_lib/Frames and Transforms/Rigid Transform  TranslationMethod=Cartesian  TranslationStandardOffset=0  TranslationLengthUnit=m  TranslationStandardAxis=+Z  TranslationCartesianOffset=[0 -a 0]  TranslationROffset=0  TranslationROffsetUnits=m  TranslationZOffset=0  TranslationZOffsetUnits=m  TranslationThetaOffset=0  TranslationThetaOffsetUnits=deg  RotationMethod=StandardAxis  RotationAngleUnits=deg  RotationStandardAxis=+Y  RotationAngle=90  RotationArbitraryAxis=[0 0 1]  FollAlignAxisA=+X  BaseAlignAxisA=+Y  FollAlignAxisB=+Y  BaseAlignAxisB=+Z  RotationSequenceAxes=FollowerAxes  RotationSequence=XYX  RotationSequenceAngles=[0 0 0]  RotationSequenceAnglesUnits=deg  RotationMatrix=[1 0 0; 0 1 0; 0 0 1]
  Rigid Transform 4.4 : sm_lib/Frames and Transforms/Rigid Transform  TranslationMethod=None  TranslationStandardOffset=0  TranslationLengthUnit=m  TranslationStandardAxis=+Z  TranslationCartesianOffset=[0 0 0]  TranslationROffset=0  TranslationROffsetUnits=m  TranslationZOffset=0  TranslationZOffsetUnits=m  TranslationThetaOffset=0  TranslationThetaOffsetUnits=deg  RotationMethod=StandardAxis  RotationAngleUnits=deg  RotationStandardAxis=+X  RotationAngle=turn4  RotationArbitraryAxis=[0 0 1]  FollAlignAxisA=+X  BaseAlignAxisA=+Y  FollAlignAxisB=+Y  BaseAlignAxisB=+Z  RotationSequenceAxes=FollowerAxes  RotationSequence=XYX  RotationSequenceAngles=[0 0 0]  RotationSequenceAnglesUnits=deg  RotationMatrix=[1 0 0; 0 1 0; 0 0 1]
  Rigid Transform3.3 : sm_lib/Frames and Transforms/Rigid Transform  TranslationMethod=Cartesian  TranslationStandardOffset=0  TranslationLengthUnit=m  TranslationStandardAxis=+Z  TranslationCartesianOffset=[0 a 0]  TranslationROffset=0  TranslationROffsetUnits=m  TranslationZOffset=0  TranslationZOffsetUnits=m  TranslationThetaOffset=0  TranslationThetaOffsetUnits=deg  RotationMethod=StandardAxis  RotationAngleUnits=deg  RotationStandardAxis=+Y  RotationAngle=90  RotationArbitraryAxis=[0 0 1]  FollAlignAxisA=+X  BaseAlignAxisA=+Y  FollAlignAxisB=+Y  BaseAlignAxisB=+Z  RotationSequenceAxes=FollowerAxes  RotationSequence=XYX  RotationSequenceAngles=[0 0 0]  RotationSequenceAnglesUnits=deg  RotationMatrix=[1 0 0; 0 1 0; 0 0 1]
  Solid_Quadrilateral : sm_lib/Body Elements/Solid  InertiaType=CalculateFromGeometry  Mass=1  MassUnits=kg  CenterOfMass=[0 0 0]  CenterOfMassUnits=m  MomentsOfInertia=[1 1 1]  MomentsOfInertiaUnits=kg*m^2  ProductsOfInertia=[1 1 1]  ProductsOfInertiaUnits=kg*m^2  DensityBased=on  Density=1000  DensityUnits=kg/m^3  DoExposeReferenceFrame=on  SerializedFrames=<Frames/>  GraphicType=FromGeometry  MarkerShape=Sphere  MarkerSize=10  GraphicVisPropType=SimpleVisualProperties  GraphicDiffuseColor=clr  GraphicSpecularColor=[0.5 0.5 0.5 1.0]  GraphicAmbientColor=[0.15 0.15 0.15 1.0]  GraphicEmissiveColor=[0.0 0.0 0.0 1.0]  GraphicShininess=75  GraphicOpacity=tr  GeometryShape=GeneralExtrusion  RectangleSize=[1 1]  RectangleSizeUnits=m  BrickDimensions=quadrilateral  BrickDimensionUnits=m  CylinderRadius=1  CylinderRadiusUnits=m  CylinderLength=1  CylinderLengthUnits=m  SphereRadius=1  SphereRadiusUnits=m  EllipsoidRadii=[1 1 1]  EllipsoidRadiiUnits=m  ExtrusionCrossSection=quadrilateral  ExtrusionCrossSectionUnits=m  ExtrusionLength=t  ExtrusionLengthUnits=m  PolygonNumSides=3  PolygonOuterRadius=1  PolygonOuterRadiusUnits=m  ExtGeomFileType=STEP  ExtGeomFileUnits=m  RevolutionCrossSection=[1 1; 1 -1; 2 -1; 2 1]  RevolutionCrossSectionUnits=m  RevolutionExtent=Full  RevolutionAngle=180  RevolutionAngleUnits=deg
  Solid_RJ1 : sm_lib/Body Elements/Solid  InertiaType=PointMass  Mass=0  MassUnits=kg  CenterOfMass=[0 0 0]  CenterOfMassUnits=m  MomentsOfInertia=[1 1 1]  MomentsOfInertiaUnits=kg*m^2  ProductsOfInertia=[1 1 1]  ProductsOfInertiaUnits=kg*m^2  DensityBased=on  Density=1000  DensityUnits=kg/m^3  DoExposeReferenceFrame=off  SerializedFrames=<Frames><Frame><Id>Frame1</Id><Value><Name>S1</Name><Origin><Source>ReferenceFrame</Source><FeatureName></FeatureName></Origin><PrimaryAxis><DefinedDirection>+Z</DefinedDirection><Source>ReferenceFrame</Source><SourceDirection>+Z</SourceDirection><FeatureName></FeatureName></PrimaryAxis><SecondaryAxis><DefinedDirection>+X</DefinedDirection><Source>ReferenceFrame</Source><SourceDirection>+X</SourceDirection><FeatureName></FeatureName></SecondaryAxis></Value></Frame></Frames>  GraphicType=FromGeometry  MarkerShape=Sphere  MarkerSize=10  GraphicVisPropType=SimpleVisualProperties  GraphicDiffuseColor=cl_joint  GraphicSpecularColor=[0.5 0.5 0.5 1.0]  GraphicAmbientColor=[0.15 0.15 0.15 1.0]  GraphicEmissiveColor=[0.0 0.0 0.0 1.0]  GraphicShininess=75  GraphicOpacity=rj_true1  GeometryShape=Cylinder  RectangleSize=[1 1]  RectangleSizeUnits=m  BrickDimensions=[1 1 1]  BrickDimensionUnits=m  CylinderRadius=t_rj  CylinderRadiusUnits=m  CylinderLength=l1  CylinderLengthUnits=m  SphereRadius=1  SphereRadiusUnits=m  EllipsoidRadii=[1 1 1]  EllipsoidRadiiUnits=m  ExtrusionCrossSection=[1 1; -1 1; -1 -1; 1 -1]  ExtrusionCrossSectionUnits=m  ExtrusionLength=1  ExtrusionLengthUnits=m  PolygonNumSides=3  PolygonOuterRadius=1  PolygonOuterRadiusUnits=m  ExtGeomFileType=STEP  ExtGeomFileUnits=m  RevolutionCrossSection=[1 1; 1 -1; 2 -1; 2 1]  RevolutionCrossSectionUnits=m  RevolutionExtent=Full  RevolutionAngle=180  RevolutionAngleUnits=deg
  Solid_RJ2 : sm_lib/Body Elements/Solid  InertiaType=PointMass  Mass=0  MassUnits=kg  CenterOfMass=[0 0 0]  CenterOfMassUnits=m  MomentsOfInertia=[1 1 1]  MomentsOfInertiaUnits=kg*m^2  ProductsOfInertia=[1 1 1]  ProductsOfInertiaUnits=kg*m^2  DensityBased=on  Density=1000  DensityUnits=kg/m^3  DoExposeReferenceFrame=off  SerializedFrames=<Frames><Frame><Id>Frame1</Id><Value><Name>S2</Name><Origin><Source>ReferenceFrame</Source><FeatureName></FeatureName></Origin><PrimaryAxis><DefinedDirection>+Z</DefinedDirection><Source>ReferenceFrame</Source><SourceDirection>+Z</SourceDirection><FeatureName></FeatureName></PrimaryAxis><SecondaryAxis><DefinedDirection>+X</DefinedDirection><Source>ReferenceFrame</Source><SourceDirection>+X</SourceDirection><FeatureName></FeatureName></SecondaryAxis></Value></Frame></Frames>  GraphicType=FromGeometry  MarkerShape=Sphere  MarkerSize=10  GraphicVisPropType=SimpleVisualProperties  GraphicDiffuseColor=cl_joint  GraphicSpecularColor=[0.5 0.5 0.5 1.0]  GraphicAmbientColor=[0.15 0.15 0.15 1.0]  GraphicEmissiveColor=[0.0 0.0 0.0 1.0]  GraphicShininess=75  GraphicOpacity=rj_true2  GeometryShape=Cylinder  RectangleSize=[1 1]  RectangleSizeUnits=m  BrickDimensions=[1 1 1]  BrickDimensionUnits=m  CylinderRadius=t_rj  CylinderRadiusUnits=m  CylinderLength=l2  CylinderLengthUnits=m  SphereRadius=1  SphereRadiusUnits=m  EllipsoidRadii=[1 1 1]  EllipsoidRadiiUnits=m  ExtrusionCrossSection=[1 1; -1 1; -1 -1; 1 -1]  ExtrusionCrossSectionUnits=m  ExtrusionLength=1  ExtrusionLengthUnits=m  PolygonNumSides=3  PolygonOuterRadius=1  PolygonOuterRadiusUnits=m  ExtGeomFileType=STEP  ExtGeomFileUnits=m  RevolutionCrossSection=[1 1; 1 -1; 2 -1; 2 1]  RevolutionCrossSectionUnits=m  RevolutionExtent=Full  RevolutionAngle=180  RevolutionAngleUnits=deg
  Solid_RJ3 : sm_lib/Body Elements/Solid  InertiaType=PointMass  Mass=0  MassUnits=kg  CenterOfMass=[0 0 0]  CenterOfMassUnits=m  MomentsOfInertia=[1 1 1]  MomentsOfInertiaUnits=kg*m^2  ProductsOfInertia=[1 1 1]  ProductsOfInertiaUnits=kg*m^2  DensityBased=on  Density=1000  DensityUnits=kg/m^3  DoExposeReferenceFrame=off  SerializedFrames=<Frames><Frame><Id>Frame1</Id><Value><Name>S3</Name><Origin><Source>ReferenceFrame</Source><FeatureName></FeatureName></Origin><PrimaryAxis><DefinedDirection>+Z</DefinedDirection><Source>ReferenceFrame</Source><SourceDirection>+Z</SourceDirection><FeatureName></FeatureName></PrimaryAxis><SecondaryAxis><DefinedDirection>+X</DefinedDirection><Source>ReferenceFrame</Source><SourceDirection>+X</SourceDirection><FeatureName></FeatureName></SecondaryAxis></Value></Frame></Frames>  GraphicType=FromGeometry  MarkerShape=Sphere  MarkerSize=10  GraphicVisPropType=SimpleVisualProperties  GraphicDiffuseColor=cl_joint  GraphicSpecularColor=[0.5 0.5 0.5 1.0]  GraphicAmbientColor=[0.15 0.15 0.15 1.0]  GraphicEmissiveColor=[0.0 0.0 0.0 1.0]  GraphicShininess=75  GraphicOpacity=rj_true3  GeometryShape=Cylinder  RectangleSize=[1 1]  RectangleSizeUnits=m  BrickDimensions=[1 1 1]  BrickDimensionUnits=m  CylinderRadius=t_rj  CylinderRadiusUnits=m  CylinderLength=l3  CylinderLengthUnits=m  SphereRadius=1  SphereRadiusUnits=m  EllipsoidRadii=[1 1 1]  EllipsoidRadiiUnits=m  ExtrusionCrossSection=[1 1; -1 1; -1 -1; 1 -1]  ExtrusionCrossSectionUnits=m  ExtrusionLength=1  ExtrusionLengthUnits=m  PolygonNumSides=3  PolygonOuterRadius=1  PolygonOuterRadiusUnits=m  ExtGeomFileType=STEP  ExtGeomFileUnits=m  RevolutionCrossSection=[1 1; 1 -1; 2 -1; 2 1]  RevolutionCrossSectionUnits=m  RevolutionExtent=Full  RevolutionAngle=180  RevolutionAngleUnits=deg
  Solid_RJ4 : sm_lib/Body Elements/Solid  InertiaType=PointMass  Mass=0  MassUnits=kg  CenterOfMass=[0 0 0]  CenterOfMassUnits=m  MomentsOfInertia=[1 1 1]  MomentsOfInertiaUnits=kg*m^2  ProductsOfInertia=[1 1 1]  ProductsOfInertiaUnits=kg*m^2  DensityBased=on  Density=1000  DensityUnits=kg/m^3  DoExposeReferenceFrame=off  SerializedFrames=<Frames><Frame><Id>Frame1</Id><Value><Name>S4</Name><Origin><Source>ReferenceFrame</Source><FeatureName></FeatureName></Origin><PrimaryAxis><DefinedDirection>+Z</DefinedDirection><Source>ReferenceFrame</Source><SourceDirection>+Z</SourceDirection><FeatureName></FeatureName></PrimaryAxis><SecondaryAxis><DefinedDirection>+X</DefinedDirection><Source>ReferenceFrame</Source><SourceDirection>+X</SourceDirection><FeatureName></FeatureName></SecondaryAxis></Value></Frame></Frames>  GraphicType=FromGeometry  MarkerShape=Sphere  MarkerSize=10  GraphicVisPropType=SimpleVisualProperties  GraphicDiffuseColor=cl_joint  GraphicSpecularColor=[0.5 0.5 0.5 1.0]  GraphicAmbientColor=[0.15 0.15 0.15 1.0]  GraphicEmissiveColor=[0.0 0.0 0.0 1.0]  GraphicShininess=75  GraphicOpacity=rj_true4  GeometryShape=Cylinder  RectangleSize=[1 1]  RectangleSizeUnits=m  BrickDimensions=[1 1 1]  BrickDimensionUnits=m  CylinderRadius=t_rj  CylinderRadiusUnits=m  CylinderLength=l4  CylinderLengthUnits=m  SphereRadius=1  SphereRadiusUnits=m  EllipsoidRadii=[1 1 1]  EllipsoidRadiiUnits=m  ExtrusionCrossSection=[1 1; -1 1; -1 -1; 1 -1]  ExtrusionCrossSectionUnits=m  ExtrusionLength=1  ExtrusionLengthUnits=m  PolygonNumSides=3  PolygonOuterRadius=1  PolygonOuterRadiusUnits=m  ExtGeomFileType=STEP  ExtGeomFileUnits=m  RevolutionCrossSection=[1 1; 1 -1; 2 -1; 2 1]  RevolutionCrossSectionUnits=m  RevolutionExtent=Full  RevolutionAngle=180  RevolutionAngleUnits=deg
  S1 : PMIOPort  Port=1  Side=Left
  S2 : PMIOPort  Port=2  Side=Left
  S3 : PMIOPort  Port=3  Side=Right
  S4 : PMIOPort  Port=4  Side=Right
  connections:
  S2/RConn1 -- Solid_RJ2/LConn1 -- Rigid Transform 2.2/RConn1
  Rigid Transform 2.2/LConn1 -- Rigid Transform 2.1/RConn1
  Rigid Transform 3.2/RConn1 -- Rigid Transform3.3/LConn1
  Rigid Transform 3.4/LConn1 -- Rigid Transform3.3/RConn1
  Rigid Transform 3.2/LConn1 -- Rigid Transform 3.1/RConn1
  Rigid Transform 4.3/LConn1 -- Rigid Transform 4.2/RConn1
  S4/RConn1 -- Solid_RJ4/LConn1 -- Rigid Transform 4.4/RConn1
  S3/RConn1 -- Solid_RJ3/LConn1 -- Rigid Transform 3.4/RConn1
  Rigid Transform 1.4/LConn1 -- Rigid Transform 1.3/RConn1
  Rigid Transform 1.4/RConn1 -- Solid_RJ1/LConn1 -- S1/RConn1
  Rigid Transform 1.3/LConn1 -- Rigid Transform 1.2/RConn1
  Rigid Transform 1.2/LConn1 -- Rigid Transform 1.1/RConn1
  Solid_Quadrilateral/RConn1 -- Rigid Transform 3.1/LConn1 -- Rigid Transform 4.1/LConn1 -- Rigid Transform 1.1/LConn1 -- Rigid Transform 2.1/LConn1
  Rigid Transform 4.3/RConn1 -- Rigid Transform 4.4/LConn1
  Rigid Transform 4.2/LConn1 -- Rigid Transform 4.1/RConn1
